simulink model "npc_controller"  (R2022a)
settings: Solver=FixedStepDiscrete  StartTime=0.0  StopTime=20  RelTol=1e-3  EnableMultiTasking=on
undefined symbols (not defined in the file): CAN_O_INT, CANA_BASE, Down, GPTRIP1SEL, GPTRIP2SEL, GPTRIP3SEL, Tsw, TZ1, TZ2, TZ3, Up
libraries: simulink x147, hdlsllib x90, c2802xlib x34, c2837xDlib x20, c280xlib x12, canmsglib x9, c2838xlib x8, idelinklib_common x3, c2806xlib x2, slpidlib x2, c28004xlib x2, c281xlib x2
(part 2 of 42)

== system npc_controller/CONTROL/CONTROL ==
  adc_in : Inport  OutDataTypeStr=Bus: adc_rect
  control_en1 : Inport  Port=2
  ref1 : Inport  Port=3
  angle1 : Inport  Port=4
  pol_pha1 : Inport  Port=5
  pol_phb1 : Inport  Port=6
  pol_phc1 : Inport  Port=7
  pha_en1 : Inport  Port=8
  phb_en1 : Inport  Port=9
  phc_en1 : Inport  Port=10
  pfc_ok2 : Inport  Port=11  OutDataTypeStr=boolean
  Trigger : TriggerPort  TriggerType=function-call  VariantControl=Variant  PortDimensions=1
  Data Store Read : DataStoreRead  DataStoreName=u8PriFutEnable  IndexOptions=Index vector (dialog)  Indices=1  OutputSizes=1
  If : If  IfExpression=u1 == 0
  false : Subsystem  TreatAsAtomicUnit=on
  sim_cmp1 : Outport
  Vpk : Outport  Port=2
  wires:
  If/1 -> false/Action
  Data Store Read/1 -> If/1
  adc_in/1 -> false/1(adc_in)
  control_en1/1 -> false/2(control_en1)
  ref1/1 -> false/3(ref1)
  false/1(sim_cmp1) -> sim_cmp1/1
  angle1/1 -> false/4(angle1)
  pol_pha1/1 -> false/5(pol_pha1)
  pol_phb1/1 -> false/6(pol_phb1)
  pol_phc1/1 -> false/7(pol_phc1)
  pha_en1/1 -> false/8(pha_en1)
  phb_en1/1 -> false/9(phb_en1)
  phc_en1/1 -> false/10(phc_en1)
  false/2(Vpk) -> Vpk/1
  pfc_ok2/1 -> false/11(pfc_ok2)

== system npc_controller/CONTROL/GET_ADC ==
  note: actual to vadc:
      | va               0.001799
      | vb               "
      | vc               "
      | vbulk          0.003623
      | vmid           0.006453
      | vaux           N/A
      |
      | icsa            0.019524
      | icsb            "
      | icsc            "
      | iphasea      0.02
      | iphaseb      "
      | iphasec      "
      |
      | tmp_mux    -
  adc_in : Inport
  Trigger : TriggerPort  TriggerType=function-call  VariantControl=Variant  PortDimensions=1
  ADC : Subsystem  Variant=on
  adc_out : Outport
  adc_rect : Outport  Port=2
  wires:
  adc_in/1 -> ADC/1(adc_in)
  ADC/1(adc_out) -> adc_out/1
  ADC/2(adc_rect) -> adc_rect/1

== system npc_controller/CONTROL/GPIO_HIGH ==
  Trigger : TriggerPort  TriggerType=function-call  VariantControl=Variant  PortDimensions=1
  Constant1 : Constant  Commented=on  OutDataTypeStr=single
  GPIO85_pin86 : c2837xDlib/Digital Output  Commented=on  GPIO_Number=GPIO80~GPIO87  GPIO_Bit0=off  GPIO_BIT0_Toggle=off  GPIO_Bit1=off  GPIO_BIT1_Toggle=off  GPIO_Bit2=off  GPIO_BIT2_Toggle=off  GPIO_Bit3=off  GPIO_BIT3_Toggle=off  GPIO_Bit4=off  GPIO_BIT4_Toggle=off  GPIO_Bit5=on  GPIO_BIT5_Toggle=off  GPIO_Bit6=off  GPIO_BIT6_Toggle=off  GPIO_Bit7=off  GPIO_BIT7_Toggle=off
      settings: SourceProductBaseCode=TIC2000
  wires:
  Constant1/1 -> GPIO85_pin86/1

== system npc_controller/CONTROL/GPIO_LOW ==
  Trigger : TriggerPort  TriggerType=function-call  VariantControl=Variant  PortDimensions=1
  Constant1 : Constant  Commented=on  Value=0  OutDataTypeStr=single
  GPIO85_pin86 : c2837xDlib/Digital Output  Commented=on  GPIO_Number=GPIO80~GPIO87  GPIO_Bit0=off  GPIO_BIT0_Toggle=off  GPIO_Bit1=off  GPIO_BIT1_Toggle=off  GPIO_Bit2=off  GPIO_BIT2_Toggle=off  GPIO_Bit3=off  GPIO_BIT3_Toggle=off  GPIO_Bit4=off  GPIO_BIT4_Toggle=off  GPIO_Bit5=on  GPIO_BIT5_Toggle=off  GPIO_Bit6=off  GPIO_BIT6_Toggle=off  GPIO_Bit7=off  GPIO_BIT7_Toggle=off
      settings: SourceProductBaseCode=TIC2000
  wires:
  Constant1/1 -> GPIO85_pin86/1

== system npc_controller/CONTROL/POLARITY ==
  note: Note:
      | 0 - pos
      | 1 - neg
  adc_in : Inport  OutDataTypeStr=Bus: adc
  Trigger : TriggerPort  TriggerType=function-call  VariantControl=Variant  PortDimensions=1
  Bus Selector : BusSelector  OutputSignals=va,vb,vc,ia,ib,ic,vbulk,vmid
  Constant : Constant  Value=0  OutDataTypeStr=single  SampleTime=-1
  Constant1 : Constant  Value=0  OutDataTypeStr=single  SampleTime=-1
  Constant2 : Constant  Value=0  OutDataTypeStr=single  SampleTime=-1
  GreaterThan : RelationalOperator  Operator=<  OutDataTypeStr=boolean  RndMeth=Simplest  InputSameDT=off
  GreaterThan1 : RelationalOperator  Operator=<  OutDataTypeStr=boolean  RndMeth=Simplest  InputSameDT=off
  GreaterThan2 : RelationalOperator  Operator=<  OutDataTypeStr=boolean  RndMeth=Simplest  InputSameDT=off
  Mux : Mux  Inputs=3
  PLL_Block1 : Subsystem  Commented=on  TreatAsAtomicUnit=on
      settings: RTWFcnNameOpts=Use subsystem name
  Scope : Scope  NumInputPorts=2
  Scope4 : Scope  Commented=on  NumInputPorts=4
  pol_pha : Outport
  pol_phb : Outport  Port=2
  pol_phc : Outport  Port=3
  wires:
  GreaterThan1/1 -> pol_phb/1
  GreaterThan/1 -> Scope/2, pol_pha/1
  adc_in/1 -> Bus Selector/1
  Bus Selector/1 -> [van]  "<va>"
  Bus Selector/3 -> [vcn]  "<vc>"
  Bus Selector/2 -> [vbn]  "<vb>"
  Constant/1 -> GreaterThan/2
  [van] -> Scope/1, GreaterThan/1
  GreaterThan2/1 -> pol_phc/1
  Constant1/1 -> GreaterThan1/2
  Constant2/1 -> GreaterThan2/2
  [vcn] -> GreaterThan2/1
  [vbn] -> GreaterThan1/1
  [van] -> Scope4/4
  [vbn] -> Scope4/2
  [van] -> Mux/3
  Mux/1 -> PLL_Block1/1(abc)
  [vcn] -> Scope4/3
  [vcn] -> Mux/2
  [vbn] -> Mux/1
  PLL_Block1/1(theta) -> Scope4/1  "va"

== system npc_controller/CONTROL/STATE-MACHINE ==
  note: States:
      | 0 - Calibraiton
      | 1 - Fault
      | 2 - FUT mode
      | 3 - NA
      | 4 - Control ON
      | 5 - Burst mode
      | 6 - PFC_EN Low
      | 7 - AC_OK Low
  note: 1 - Leg A
      | 2 - Leg B
      | 3 - Leg C
      | 4 - All legs
  note: 0 - Three phase
      | 1 - Single phase
  adc_out : Inport
  Vpk : Inport  Port=2
  Trigger : TriggerPort  TriggerType=function-call  VariantControl=Variant  PortDimensions=1
  Add : Sum  Commented=on  Inputs=+-  AccumDataTypeStr=single  OutDataTypeStr=single
  Bus Selector : BusSelector  OutputSignals=va,vb,vc,ia,ib,ic,vbulk,vmid
  CPU_CONTROL_100_A2_precharge_pfc_ok2 : Stateflow chart  Commented=on  TreatAsAtomicUnit=on
  CPU_CONTROL_200_A2_precharge_pfc_ok2 : Stateflow chart  Commented=on  TreatAsAtomicUnit=on
  CPU_CONTROL_200_A2_precharge_pfc_ok2_OL SS : Stateflow chart  Commented=on  TreatAsAtomicUnit=on
  CPU_CONTROL_200_A2_precharge_pfc_ok2_OL SS1 : Stateflow chart  Commented=on  TreatAsAtomicUnit=on
  CPU_CONTROL_200_Vpk : Stateflow chart  Commented=on  TreatAsAtomicUnit=on
  CPU_CONTROL_400 : Stateflow chart  Commented=on  TreatAsAtomicUnit=on
  CPU_CONTROL_400_A2_precharge_pfc_ok2_OL SS : Stateflow chart  Commented=on  TreatAsAtomicUnit=on
  CPU_CONTROL_750_A2_precharge_pfc_ok1 : Stateflow chart  Commented=on  TreatAsAtomicUnit=on
  CPU_CONTROL_750_A2_precharge_pfc_ok2_OL SS1 : Stateflow chart  Commented=on  TreatAsAtomicUnit=on
  CPU_CONTROL_750_A2_precharge_pfc_ok2_OL SS2 : Stateflow chart  TreatAsAtomicUnit=on
  CPU_CONTROL_750_Vpk : Stateflow chart  Commented=on  TreatAsAtomicUnit=on
  CPU_CONTROL_750_precharge_pfc_ok2 : Stateflow chart  Commented=on  TreatAsAtomicUnit=on
  Cast To Single : DataTypeConversion  Commented=on  OutDataTypeStr=uint16  SaturateOnIntegerOverflow=off  RndMeth=Floor
  Cast To Single1 : DataTypeConversion  Commented=on  OutDataTypeStr=single  SaturateOnIntegerOverflow=off  RndMeth=Floor
  Cast To Single2 : DataTypeConversion  OutDataTypeStr=single  SaturateOnIntegerOverflow=off  RndMeth=Floor
  Cast To Single3 : DataTypeConversion  Commented=on  OutDataTypeStr=single  SaturateOnIntegerOverflow=off  RndMeth=Floor
  Constant : Constant  OutDataTypeStr=boolean
  Constant2 : Constant  Commented=on  Value=200  OutDataTypeStr=single
  DAC : c2837xDlib/DAC  Commented=on  channel=B  saturate=on
      settings: SourceProductBaseCode=TIC2000
  Data Store Read : DataStoreRead  Commented=on  DataStoreName=debug_en  IndexOptions=Index vector (dialog)  Indices=1  OutputSizes=1
  Data Store Read1 : DataStoreRead  DataStoreName=u8PriFutEnable  IndexOptions=Index vector (dialog)  Indices=1  OutputSizes=1
  Data Store Read2 : DataStoreRead  DataStoreName=u8GridPhaseType  IndexOptions=Index vector (dialog)  Indices=1  OutputSizes=1
  Data Store Read3 : DataStoreRead  DataStoreName=u8SinglePhaseLeg  IndexOptions=Index vector (dialog)  Indices=1  OutputSizes=1
  Data Store Read4 : DataStoreRead  DataStoreName=pfc_en  IndexOptions=Index vector (dialog)  Indices=1  OutputSizes=1
  Data Store Read5 : DataStoreRead  DataStoreName=rms_vc  IndexOptions=Index vector (dialog)  Indices=1  OutputSizes=1
  Data Store Write : DataStoreWrite  DataStoreName=u16Debug1  IndexOptions=Index vector (dialog)  Indices=1  OutputSizes=1
  Data Store Write12 : DataStoreWrite  DataStoreName=relay_ctrl  IndexOptions=Index vector (dialog)  Indices=1  OutputSizes=1
  Data Store Write13 : DataStoreWrite  DataStoreName=pfc_ok  IndexOptions=Index vector (dialog)  Indices=1  OutputSizes=1
  Data Store Write3 : DataStoreWrite  DataStoreName=ac_ok  IndexOptions=Index vector (dialog)  Indices=1  OutputSizes=1
  Data Store Write4 : DataStoreWrite  DataStoreName=pfc_en  IndexOptions=Index vector (dialog)  Indices=1  OutputSizes=1
  Data Store Write5 : DataStoreWrite  Commented=on  DataStoreName=Vbulk_Ref  IndexOptions=Index vector (dialog)  Indices=1  OutputSizes=1
  Digital Output : c2837xDlib/Digital Output  Commented=on  GPIO_Number=GPIO136~GPIO143  GPIO_Bit0=off  GPIO_BIT0_Toggle=off  GPIO_Bit1=off  GPIO_BIT1_Toggle=off  GPIO_Bit2=off  GPIO_BIT2_Toggle=off  GPIO_Bit3=on  GPIO_BIT3_Toggle=off  GPIO_Bit4=off  GPIO_BIT4_Toggle=off  GPIO_Bit5=off  GPIO_BIT5_Toggle=off  GPIO_Bit6=off  GPIO_BIT6_Toggle=off  GPIO_Bit7=off  GPIO_BIT7_Toggle=off
      settings: SourceProductBaseCode=TIC2000
  Gain : Gain  Commented=on  Gain=4095/831.7167
  Gain1 : Gain  Commented=on  Gain=2000  ParamDataTypeStr=single  OutDataTypeStr=single
  Gain2 : Gain  Gain=500  ParamDataTypeStr=single  OutDataTypeStr=single
  Gain3 : Gain  Gain=1.414  OutDataTypeStr=single
  If : If  Commented=on  IfExpression=u1 == 0
  If Action Subsystem : Subsystem  Commented=on  TreatAsAtomicUnit=on
  If Action Subsystem1 : Subsystem  Commented=on  TreatAsAtomicUnit=on
  Merge : Merge  Commented=on
  NOT : Logic  Operator=NOT  IconShape=distinctive  AllPortsSameDT=off  OutDataTypeStr=boolean
  PFC_EN_GPIO60 : c2837xDlib/Digital Input  GPIO_Number=GPIO56~GPIO63  GPIO_Bit0=off  GPIO_Bit1=off  GPIO_Bit2=off  GPIO_Bit3=off  GPIO_Bit4=on  GPIO_Bit5=off  GPIO_Bit6=off  GPIO_Bit7=off  sampleTime=-1  dataType=auto  GPIO_Bit0_Qualification=Sync to SYSCLKOUT  GPIO_Bit1_Qualification=Sync to SYSCLKOUT  GPIO_Bit2_Qualification=Sync to SYSCLKOUT  GPIO_Bit3_Qualification=Sync to SYSCLKOUT  GPIO_Bit4_Qualification=Sync to SYSCLKOUT  GPIO_Bit5_Qualification=Sync to SYSCLKOUT  GPIO_Bit6_Qualification=Sync to SYSCLKOUT  GPIO_Bit7_Qualification=Sync to SYSCLKOUT  Qualification_Period=-1
      settings: SourceProductBaseCode=TIC2000
  PLL : Subsystem  Commented=on
  Sin2 : Trigonometry  Commented=on  OutputSignalType=real
  Subsystem1 : Subsystem  Commented=on
  Update_PFC_EN : Subsystem
  calib_ok : Outport
  control_en : Outport  Port=2
  burst_en : Outport  Port=3
  eoss : Outport  Port=4
  ref : Outport  Port=5
  mag : Outport  Port=6
  angle : Outport  Port=7
  freq : Outport  Port=8
  va_seq : Outport  Port=9
  vb_seq : Outport  Port=10
  vc_seq : Outport  Port=11
  pha_en : Outport  Port=12
  phb_en : Outport  Port=13
  phc_en : Outport  Port=14
  pfc_ok1 : Outport  Port=15
  wires:
  CPU_CONTROL_750_A2_precharge_pfc_ok2_OL SS2/6(ref) -> ref/1, Cast To Single/1
  adc_out/1 -> Bus Selector/1
  Bus Selector/7 -> CPU_CONTROL_750_A2_precharge_pfc_ok2_OL SS2/7(vbulk)  "<vbulk>"
  Bus Selector/1 -> CPU_CONTROL_750_A2_precharge_pfc_ok2_OL SS2/1(van)  "<va>"
  Bus Selector/2 -> CPU_CONTROL_750_A2_precharge_pfc_ok2_OL SS2/2(vbn)  "<vb>"
  Bus Selector/3 -> CPU_CONTROL_750_A2_precharge_pfc_ok2_OL SS2/3(vcn)  "<vc>"
  CPU_CONTROL_750_A2_precharge_pfc_ok2_OL SS2/3(control_en) -> control_en/1
  CPU_CONTROL_750_A2_precharge_pfc_ok2_OL SS2/4(burst_en) -> burst_en/1
  CPU_CONTROL_750_A2_precharge_pfc_ok2_OL SS2/5(eoss) -> eoss/1
  Bus Selector/4 -> CPU_CONTROL_750_A2_precharge_pfc_ok2_OL SS2/4(ia)  "<ia>"
  Bus Selector/5 -> CPU_CONTROL_750_A2_precharge_pfc_ok2_OL SS2/5(ib)  "<ib>"
  Bus Selector/6 -> CPU_CONTROL_750_A2_precharge_pfc_ok2_OL SS2/6(ic)  "<ic>"
  Sin2/1 -> Subsystem1/1(adc)
  Add/1 -> PLL/1(vxn)
  Cast To Single3/1 -> Add/1
  Merge/1 -> Add/2
  PLL/2(angle) -> Sin2/1
  Subsystem1/1(adc_rect) -> angle/1  "va"
  CPU_CONTROL_750_A2_precharge_pfc_ok2_OL SS2/2(calib_ok) -> calib_ok/1
  If/1 -> If Action Subsystem1/Action
  If Action Subsystem/1(Out1) -> Merge/2
  If Action Subsystem1/1(Out1) -> Merge/1
  If/2 -> If Action Subsystem/Action
  Data Store Read/1 -> ?
  Data Store Read1/1 -> CPU_CONTROL_750_A2_precharge_pfc_ok2_OL SS2/8(fut_en_req)
  CPU_CONTROL_750_A2_precharge_pfc_ok2_OL SS2/10(pha_en) -> va_seq/1, pha_en/1
  CPU_CONTROL_750_A2_precharge_pfc_ok2_OL SS2/11(phb_en) -> vb_seq/1, phb_en/1
  CPU_CONTROL_750_A2_precharge_pfc_ok2_OL SS2/12(phc_en) -> vc_seq/1, phc_en/1
  CPU_CONTROL_750_A2_precharge_pfc_ok2_OL SS2/1(state) -> Data Store Write/1, Cast To Single2/1
  Cast To Single/1 -> ?
  Data Store Read2/1 -> CPU_CONTROL_750_A2_precharge_pfc_ok2_OL SS2/9(grid_config_req)
  Data Store Read3/1 -> CPU_CONTROL_750_A2_precharge_pfc_ok2_OL SS2/10(singleph_config_req)
  Cast To Single1/1 -> Gain1/1
  Cast To Single2/1 -> Gain2/1
  Gain2/1 -> ?
  Data Store Read5/1 -> Gain3/1
  CPU_CONTROL_750_A2_precharge_pfc_ok2_OL SS2/13(pfc_ok) -> pfc_ok1/1, Data Store Write13/1
  CPU_CONTROL_750_A2_precharge_pfc_ok2_OL SS2/14(relay_ctrl) -> Data Store Write12/1
  Data Store Read4/1 -> CPU_CONTROL_750_A2_precharge_pfc_ok2_OL SS2/12(pfc_en)
  CPU_CONTROL_750_A2_precharge_pfc_ok2_OL SS2/15(tfv_v_UvpOvp) -> NOT/1
  NOT/1 -> Data Store Write3/1
  Update_PFC_EN/1(Dig_Input_State) -> Digital Output/1, Data Store Write4/1
  Gain/1 -> Data Store Write5/1
  Constant2/1 -> Gain/1
  Gain3/1 -> CPU_CONTROL_750_A2_precharge_pfc_ok2_OL SS2/11(Vpk)
  Gain1/1 -> DAC/1
  Constant/1 -> Update_PFC_EN/1(Dig_Input)

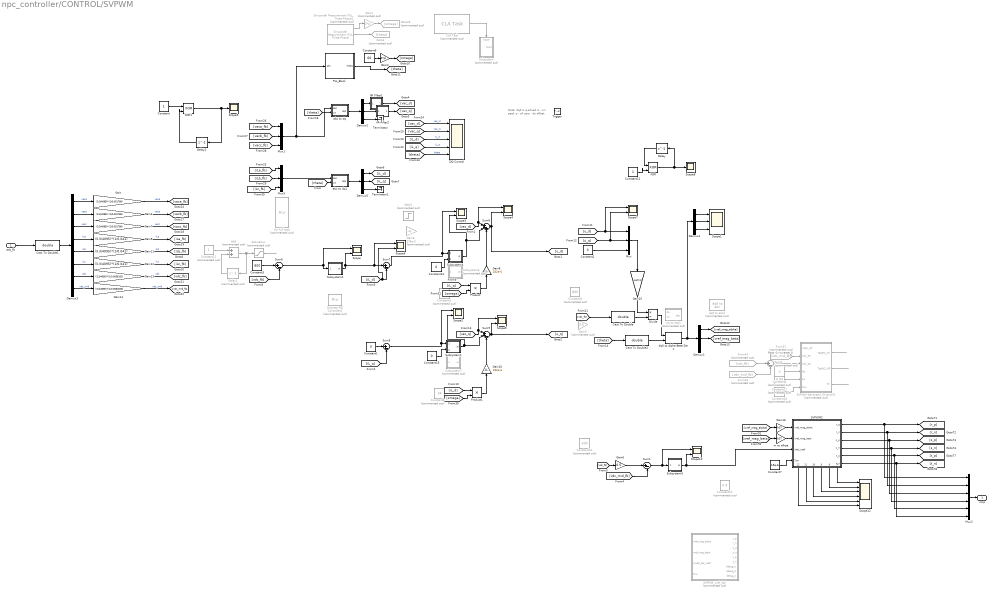
== system npc_controller/CONTROL/SVPWM ==
  note: Note: dq0 is q-alined
      | d - vin peak
      | q - pf
      | zero - dc offset
  note: Rect -1, inverter 0
  adc_fb : Inport
  Trigger : TriggerPort  TriggerType=function-call  VariantControl=Variant  PortDimensions=1
  Add : Sum  Commented=on
  CLA Task : c2806xlib/CLA Task  Commented=on  taskNumber=1  intSource=Software  wait=off  sampleTime=-1  claType=0  softTrigSelected=1  enableInterrupt=on
      settings: SourceProductName=Embedded Coder Support Package for Texas Instruments C2000 Processors
  Cast To Double : DataTypeConversion  OutDataTypeStr=double  SaturateOnIntegerOverflow=off  RndMeth=Floor
  Cast To Double1 : DataTypeConversion  OutDataTypeStr=double  SaturateOnIntegerOverflow=off  RndMeth=Floor
  Cast To Double2 : DataTypeConversion  OutDataTypeStr=double  SaturateOnIntegerOverflow=off  RndMeth=Floor
  Constant : Constant
  Constant{1..2,13,15} (4 alike) : Constant  Value=0
  Constant10 : Constant  Commented=on  Value=0.9
  Constant11 : Constant  Commented=on
  Constant12 : Constant
  Constant14 : Constant  Commented=on  Value=400
  Constant17 : Constant  Commented=on  Value=0.04
  Constant18 : Constant  Commented=on  Value=65e3
  Constant3 : Constant  Value=800
  Constant4 : Constant  Commented=on  Value=-1
  Constant5 : Constant  Commented=on  Value=34
  Constant6 : Constant  Value=60
  Constant7 : Constant  Value=15e-6
  Constant8 : Constant  Commented=on  Value=34
  Constant9 : Constant  Commented=on  Value=800
  DQ Control : Scope  NumInputPorts=5
  Delay : Delay  DelayLength=1
  Delay1 : Delay  Commented=on  DelayLength=1
  Delay2 : Delay  DelayLength=1
  Demux{1..2,4..5} (4 alike) : Demux  Outputs=3
  Demux3 : Demux  Outputs=8
  Discrete PID Controller2 : slpidlib/PID Controller  Commented=on  Controller=PI  Form=Ideal  TimeDomain=Discrete-time  UseExternalTs=off  SampleTime=-1  IntegratorMethod=Forward Euler  FilterMethod=Forward Euler  ControllerParametersSource=internal  P=0.611  I=33.333  UseKiTs=off  D=0  N=100  UseFilter=on  TunerSelectOption=Transfer Function Based (PID Tuner App)  InitialConditionSource=internal  InitialConditionForIntegrator=22  InitialConditionForFilter=0  DifferentiatorICPrevScaledInput=0  ExternalReset=none  TrackingMode=off  Kt=1  LimitOutput=on  SatLimitsSource=internal  UpperSaturationLimit=36  LowerSaturationLimit=-36  LinearizeAsGain=off  AntiWindupMode=none  Kb=1  POutMin=[]  POutMax=[]  IOutMin=[]  IOutMax=[]  DOutMin=[]  DOutMax=[]  NOutMin=[]  NOutMax=[]  SumOutMin=[]  SumOutMax=[]  SaturationOutMin=[]  SaturationOutMax=[]  PParamMin=[]  PParamMax=[]  IParamMin=[]  IParamMax=[]  DParamMin=[]  DParamMax=[]  NParamMin=[]  NParamMax=[]  KbParamMin=[]  KbParamMax=[]  KtParamMin=[]  KtParamMax=[]  KbOutMin=[]  KbOutMax=[]  KtOutMin=[]  KtOutMax=[]  IntegratorOutMin=[]  IntegratorOutMax=[]  FilterOutMin=[]  FilterOutMax=[]  SumI1OutMin=[]  SumI1OutMax=[]  SumI2OutMin=[]  SumI2OutMax=[]  SumI3OutMin=[]  SumI3OutMax=[]  SumI4OutMin=[]  SumI4OutMax=[]  SumDOutMin=[]  SumDOutMax=[]  DifferentiatorOutMin=[]  DifferentiatorOutMax=[]  FilterDiffOutCoefMin=[]  FilterDiffOutCoefMax=[]  ReciprocalOutMin=[]  ReciprocalOutMax=[]  SumDenOutMin=[]  SumDenOutMax=[]  SumNumOutMin=[]  SumNumOutMax=[]  DivideOutMin=[]  DivideOutMax=[]  UdiffTsProdOutMin=[]  UdiffTsProdOutMax=[]  NTsProdOutMin=[]  NTsProdOutMax=[]  UintegralTsProdOutMin=[]  UintegralTsProdOutMax=[]  UngainTsProdOutMin=[]  UngainTsProdOutMax=[]  IntegratorContinuousStateAttributes=''  IntegratorStateMustResolveToSignalObject=off  IntegratorRTWStateStorageClass=Auto  FilterContinuousStateAttributes=''  FilterStateMustResolveToSignalObject=off  FilterRTWStateStorageClass=Auto  ParallelPVariant=Passthrough  IdealPVariant=InternalParameters  IVariant=InternalParameters  DVariant=Disabled  IntegratorVariant=Discrete  SatVariant=Enabled  AWVariant=Passthrough  PCopyVariant=Disabled  TRVariant=Disabled  FdbkBlocksVariant=Forward  IdealPFdbkVariant=Disabled  SatFdbkVariant=Disabled  DerivativeFilterVariant=Disabled  NVariant=Disabled  NCopyVariant=Disabled_SignalSpec  FilterICVariant=Disabled  IntegratorICVariant=InternalICs  ExternalResetVariant=Disabled  TRSumVariant=Passthrough  SumFdbkVariant=Disabled  SumVariant=Sum_PI  TsampFilterVariant=InternalTs  TsampNgainVariant=Passthrough  TsampIntegralVariant=Passthrough  ExternalSaturationOutDataTypeStr=Inherit: Same as second input  aMode=0
  Divide : Product  Inputs=*/
  From37 : From  Commented=on  GotoTag=vdc_mid_fb
  From42 : From  Commented=on  GotoTag=vdc_mid_fb
  From43 : From  Commented=on  GotoTag=vdc_fb
  Gain : Gain  Gain=(3.3/4095)*(1/0.001798)
  Gain1 : Gain  Commented=on  Gain=2*pi
  Gain10 : Gain  Gain=182e-6
  Gain11 : Gain  Gain=(3.3/4095)*(1/0.041)
  Gain12 : Gain  Gain=(3.3/4095)*(1/0.041)
  Gain13 : Gain  Gain=(3.3/4095)*(1/0.0036102)
  Gain14 : Gain  Gain=(3.3/4095)*(1/0.0064528)
  Gain15 : Gain  Gain=sqrt(3)
  Gain16 : Gain  Gain=0.57
  Gain2 : Gain  Gain=2*pi
  Gain3 : Gain  Commented=on  Gain=2*5e-3
  Gain4 : Gain  Gain=(3.3/4095)*(1/0.001798)
  Gain5 : Gain  Commented=on  Gain=0.5
  Gain6 : Gain  Gain=0.5
  Gain7 : Gain  Gain=(3.3/4095)*(1/0.001798)
  Gain8 : Gain  Gain=182e-6
  Gain9 : Gain  Gain=(3.3/4095)*(1/0.041)
  Goto25 : Goto  Commented=on  GotoTag=omega
  Goto3 : Goto  Commented=on  GotoTag=theta
  IIR Filter1 : Subsystem
  IIR Filter2 : Subsystem
  Mux : Mux  Inputs=3
  Mux1 : Mux  Inputs=3
  Mux2 : Mux  Inputs=6
  Mux5 : Mux  Inputs=3
  PLL_Block : Subsystem  TreatAsAtomicUnit=on
      settings: RTWFcnNameOpts=Use subsystem name
  Product : Product
  Product1 : Product
  SVPWM Generator (3-Level)1 : Subsystem  Commented=on
  SVPWM2 : Stateflow chart  TreatAsAtomicUnit=on
      settings: PortSchema="{\"entries\":[{\"content\":{\"sides\":[{\"content\":{\"connectorIds\":[\"In1\",\"In2\",\"In3\",\"In4\"]},\"type\":\"ConnectorPlacement.EquallySpacedRectSide\",\"uuid\":\"7e4e3e66-8524-4070-820d-e987ee6a426b\"},{\"content\":{\"connectorIds\":[\"Out1\",\"Out2\",\"Out3\",\"Out4\",\"Out5\",\"Out6\"],\"side\":\"RIGHT\"},\"type\":\"ConnectorPlacement.EquallySpacedRectSide\",\"uuid\":\"f5c3bbe2-d26b-4560-8bc2-49e1d2ba310c\"},{\"content\":{\"connectorIds\":[],\"side\":\"TOP\"},\"type\":\"ConnectorPlacement.EquallySpacedRectSide\",\"uuid\":\"83d02455-8012-4bd6-97d4-4ddb2b0da207\"},{\"content\":{\"connectorIds\":[\"Out12\",\"Out11\",\"Out10\",\"Out9\",\"Out8\",\"Out7\"],\"side\":\"BOTTOM\"},\"type\":\"ConnectorPlacement.EquallySpacedRectSide\",\"uuid\":\"82480829-29a6-4c64-92d2-d0891a7cd2c4\"},{\"content\":{\"connectorIds\":[],\"side\":\"HIDDEN\"},\"type\":\"ConnectorPlacement.EquallySpacedRectSide\",\"uuid\":\"daebbe37-e4fd-4cc7-9cba-3ce58bd0f8bb\"}]},\"type\":\"ConnectorPlacement.EquallySpacedConnector\",\"uuid\":\"3945a731-6436-4370-b05f-e1cd706c7526\"}],\"packageUris\":[\"http://schema.mathworks.com/mf0/Connector/R2020b\"],\"version\":\"1.0\"}"
  SVPWM_with_bal : Stateflow chart  Commented=on  TreatAsAtomicUnit=on
  Saturation : Saturate  Commented=on  UpperLimit=800  LowerLimit=0
  Scope{,2..7,10} (8 alike) : Scope  NumInputPorts=2
  Scope1 : Scope  NumInputPorts=3
  Scope12 : Scope  NumInputPorts=6
  Scope8 : Scope
  Scope9 : Scope
  "Sinusoidal Measurement (PLL, Three-Phase)1" : eeSinusoidalMeasurementV2/Sinusoidal Measurement (PLL, Three-Phase)  Commented=on  Kp_LF=2  Ki_LF=20  F0=60  Theta0=0  Ts=-1
      settings: SourceProductBaseCode=PS
  Step2 : Step  Commented=on  Time=0.07  Before=10  After=2*5e-3  SampleTime=0
  Subsystem : Subsystem  Commented=on
  Subsystem1 : Subsystem
      mask Display: disp('PID(z)')
  Subsystem2 : Subsystem
      mask Display: disp('PID(z)')
  Subsystem4 : Subsystem
      mask Display: disp('PID(z)')
  Subsystem5 : Subsystem
      mask Display: disp('PID(z)')
  Subsystem6 : Subsystem  Commented=on
      mask Display: disp('PID(z)')
  Subsystem7 : Subsystem  Commented=on
      mask Display: disp('PID(z)')
  Sum{1,5..7} (4 alike) : Sum  Inputs=|+-
  Sum2 : Sum  Commented=on  Inputs=|+-
  Sum8 : Sum  Inputs=|+-+
  Sum9 : Sum  Inputs=|+--
  Terminator : Terminator
  Terminator1 : Terminator
  XOR : Logic  Operator=XOR  IconShape=distinctive  AllPortsSameDT=off  OutDataTypeStr=boolean
  XOR1 : Logic  Operator=XOR  IconShape=distinctive  AllPortsSameDT=off  OutDataTypeStr=boolean
  abc to dq : Subsystem
  abc to dq1 : Subsystem
  dq to abc2 : Subsystem  Commented=on
  dq0 to Alpha-Beta-Zero : spsdq0toAlphaBetaZeroLib/dq0 to Alpha-Beta-Zero  Alignment=90 degrees behind phase A axis
      settings: SourceProductBaseCode=PS
  dq0 to abc1 : spsdq0toabcLib/dq0 to abc  Commented=on  Alignment=90 degrees behind phase A axis
  for full load : slpidlib/PID Controller  Commented=on  Controller=PI  Form=Parallel  TimeDomain=Discrete-time  UseExternalTs=off  SampleTime=-1  IntegratorMethod=Forward Euler  FilterMethod=Forward Euler  ControllerParametersSource=internal  P=10  I=10  UseKiTs=off  D=0  N=100  UseFilter=off  TunerSelectOption=Transfer Function Based (PID Tuner App)  InitialConditionSource=internal  InitialConditionForIntegrator=0  InitialConditionForFilter=0  DifferentiatorICPrevScaledInput=0  ExternalReset=none  TrackingMode=off  Kt=1  LimitOutput=on  SatLimitsSource=external  UpperSaturationLimit=450  LowerSaturationLimit=-450  LinearizeAsGain=on  AntiWindupMode=clamping  Kb=1  POutMin=[]  POutMax=[]  IOutMin=[]  IOutMax=[]  DOutMin=[]  DOutMax=[]  NOutMin=[]  NOutMax=[]  SumOutMin=[]  SumOutMax=[]  SaturationOutMin=[]  SaturationOutMax=[]  PParamMin=[]  PParamMax=[]  IParamMin=[]  IParamMax=[]  DParamMin=[]  DParamMax=[]  NParamMin=[]  NParamMax=[]  KbParamMin=[]  KbParamMax=[]  KtParamMin=[]  KtParamMax=[]  KbOutMin=[]  KbOutMax=[]  KtOutMin=[]  KtOutMax=[]  IntegratorOutMin=[]  IntegratorOutMax=[]  FilterOutMin=[]  FilterOutMax=[]  SumI1OutMin=[]  SumI1OutMax=[]  SumI2OutMin=[]  SumI2OutMax=[]  SumI3OutMin=[]  SumI3OutMax=[]  SumI4OutMin=[]  SumI4OutMax=[]  SumDOutMin=[]  SumDOutMax=[]  DifferentiatorOutMin=[]  DifferentiatorOutMax=[]  FilterDiffOutCoefMin=[]  FilterDiffOutCoefMax=[]  ReciprocalOutMin=[]  ReciprocalOutMax=[]  SumDenOutMin=[]  SumDenOutMax=[]  SumNumOutMin=[]  SumNumOutMax=[]  DivideOutMin=[]  DivideOutMax=[]  UdiffTsProdOutMin=[]  UdiffTsProdOutMax=[]  NTsProdOutMin=[]  NTsProdOutMax=[]  UintegralTsProdOutMin=[]  UintegralTsProdOutMax=[]  UngainTsProdOutMin=[]  UngainTsProdOutMax=[]  IntegratorContinuousStateAttributes=''  IntegratorStateMustResolveToSignalObject=off  IntegratorRTWStateStorageClass=Auto  FilterContinuousStateAttributes=''  FilterStateMustResolveToSignalObject=off  FilterRTWStateStorageClass=Auto  ParallelPVariant=InternalParameters  IdealPVariant=Disabled  IVariant=InternalParameters  DVariant=Disabled  IntegratorVariant=Discrete  SatVariant=External  AWVariant=DiscClampingParallel  PCopyVariant=Disabled  TRVariant=Disabled  FdbkBlocksVariant=Forward  IdealPFdbkVariant=Disabled  SatFdbkVariant=Disabled  DerivativeFilterVariant=Disabled  NVariant=Disabled  NCopyVariant=Disabled_SignalSpec  FilterICVariant=Disabled  IntegratorICVariant=InternalICs  ExternalResetVariant=Disabled  TRSumVariant=Passthrough  SumFdbkVariant=Disabled  SumVariant=Sum_PI  TsampFilterVariant=InternalTs  TsampNgainVariant=Passthrough  TsampIntegralVariant=Passthrough  ExternalSaturationOutDataTypeStr=Inherit: Same as second input  aMode=0
  m to alhpa : Gain  Gain=0.57
  cmp : Outport
  wires:
  CLA Task/1 -> Subsystem/Trigger
  IIR Filter2/1(y[n]) -> [vac_q]
  IIR Filter1/1(y[n]) -> [vac_d]
  Constant15/1 -> Subsystem1/2(disable)
  Constant13/1 -> Subsystem4/2(disable)
  m to alhpa/1 -> SVPWM2/2(vref_mag_beta)
  Gain16/1 -> SVPWM2/1(vref_mag_alpha)
  Gain15/1 -> Divide/1
  Subsystem5/1(pi) -> Scope10/2, SVPWM2/3(vbal_coef)
  [vdc_fb] -> Gain6/1
  Constant7/1 -> SVPWM2/4(Tsw)
  [vdc_fb] -> Cast To Double/1
  Saturation/1 -> ?
  Delay1/1 -> Add/2
  Add/1 -> Delay1/1, Saturation/1
  Constant11/1 -> Add/1
  SVPWM2/12(debug_f) -> Scope12/6
  SVPWM2/10(debug_d) -> Scope12/4
  SVPWM2/11(debug_e) -> Scope12/5
  SVPWM2/9(debug_c) -> Scope12/3
  SVPWM2/8(debug_b) -> Scope12/2
  SVPWM2/7(debug_a) -> Scope12/1
  Gain6/1 -> Sum1/1
  Sum1/1 -> Subsystem5/1(error), Scope10/1
  [vdc_mid_fb] -> Sum1/2
  Mux2/1 -> cmp/1
  Cast To Double2/1 -> dq0 to Alpha-Beta-Zero/2
  Demux1/2 -> [vref_mag_beta]
  Demux1/1 -> [vref_mag_alpha]
  SVPWM2/2(r_n) -> [r_n], Mux2/2
  SVPWM2/3(s_p) -> [s_p], Mux2/3
  SVPWM2/5(t_p) -> [t_p], Mux2/5
  SVPWM2/6(t_n) -> [t_n], Mux2/6
  SVPWM2/4(s_n) -> [s_n], Mux2/4
  SVPWM2/1(r_p) -> [r_p], Mux2/1
  [vref_mag_beta] -> m to alhpa/1
  [vref_mag_alpha] -> Gain16/1
  Constant6/1 -> Gain2/1
  PLL_Block/1(theta) -> [theta]
  Gain2/1 -> [omega]
  abc to dq/1(dq0) -> Demux2/1
  Demux3/5 -> Gain11/1  "iLb"
  Demux3/4 -> Gain9/1  "iLa"
  Demux3/3 -> Gain7/1  "vacc"
  Demux3/2 -> Gain4/1  "vacb"
  Demux3/6 -> Gain12/1  "iLc"
  Demux3/7 -> Gain13/1  "vdc"
  Demux3/8 -> Gain14/1  "vdc_mid"
  Demux3/1 -> Gain/1  "vaca"
  Delay2/1 -> XOR1/2
  XOR1/1 -> Delay2/1, Scope9/1
  Constant/1 -> XOR1/1
  Gain14/1 -> [vdc_mid_fb]  "vdc_mid"
  Gain13/1 -> [vdc_fb]  "vdc"
  Gain12/1 -> [iLc_fb]  "iLc"
  Gain11/1 -> [iLb_fb]  "iLb"
  Gain9/1 -> [iLa_fb]  "iLa"
  Gain7/1 -> [vacc_fb]  "vacc"
  Gain4/1 -> [vacb_fb]  "vacb"
  Gain/1 -> [vaca_fb]  "vaca"
  Cast To Double1/1 -> Demux3/1
  Cast To Double/1 -> Divide/2
  SVPWM Generator (3-Level)1/3(Sn) -> ?
  SVPWM Generator (3-Level)1/2(TgABC_Off) -> ?
  SVPWM Generator (3-Level)1/1(TgABC_On) -> ?
  Sum2/1 -> SVPWM Generator (3-Level)1/3(Vdc_0N)
  From42/1 -> Sum2/2
  From37/1 -> SVPWM Generator (3-Level)1/2(Vdc_P0)
  From43/1 -> Sum2/1
  Constant17/1 -> SVPWM Generator (3-Level)1/5(Kp)
  Constant4/1 -> SVPWM Generator (3-Level)1/4(Idc)
  Constant18/1 -> SVPWM Generator (3-Level)1/6(Fsw)
  Gain1/1 -> Goto25/1
  "Sinusoidal Measurement (PLL, Three-Phase)1"/1 -> Gain1/1
  adc_fb/1 -> Cast To Double1/1
  [iLa_fb] -> Mux5/1
  [iLc_fb] -> Mux5/3
  [iLb_fb] -> Mux5/2
  [vacb_fb] -> Mux1/2
  [vaca_fb] -> Mux1/1
  [vacc_fb] -> Mux1/3
  [vac_q] -> DQ Control/2  "vac_q"
  [theta] -> DQ Control/5  "theta"
  [vac_d] -> DQ Control/1  "vac_d"
  Demux5/3 -> Terminator1/1
  [iL_d] -> DQ Control/3  "iL_d"
  [iL_q] -> DQ Control/4  "iL_q"
  Mux1/1 -> abc to dq/1(abc), PLL_Block/1(abc)
  [theta] -> abc to dq/2(wt)
  Mux5/1 -> abc to dq1/1(abc)
  Demux2/2 -> IIR Filter2/1(x[n])
  Demux5/1 -> [iL_d]
  [theta] -> abc to dq1/2(wt)
  Demux2/1 -> IIR Filter1/1(x[n])
  Demux2/3 -> Terminator/1
  Demux5/2 -> [iL_q]
  "Sinusoidal Measurement (PLL, Three-Phase)1"/2 -> Goto3/1
  abc to dq1/1(dq0) -> Demux5/1
  Gain10/1 -> Sum9/3
  Gain8/1 -> Sum8/3
  Mux/1 -> Gain15/1
  Delay/1 -> XOR/1
  XOR/1 -> Scope8/1, Delay/1
  Constant12/1 -> XOR/2
  Divide/1 -> dq0 to Alpha-Beta-Zero/1
  Subsystem2/1(pi) -> Scope/2, Sum7/1, Scope6/1
  dq0 to Alpha-Beta-Zero/1 -> Demux1/1, Demux4/1
  [theta] -> Cast To Double2/1
  [omega] -> Product1/2
  [omega] -> Product/2
  Product1/1 -> Gain10/1
  Product/1 -> Gain8/1
  [iL_q] -> Product/1
  [iL_d] -> Product1/1
  Sum9/1 -> Scope5/2, [u_q]
  Sum8/1 -> Scope4/2, [u_d]
  Constant2/1 -> Mux/3
  Demux4/3 -> Scope1/3
  Demux4/2 -> Scope1/2
  Demux4/1 -> Scope1/1
  [iL_d] -> Sum7/2, Scope6/2
  Sum5/1 -> Scope2/1, Subsystem1/1(error)
  Constant1/1 -> Sum5/1
  [iL_q] -> Sum5/2
  [vac_q] -> Sum9/1, Scope5/1
  Constant3/1 -> Sum6/1
  Sum6/1 -> Scope/1, Subsystem2/1(error)
  Subsystem4/1(pi) -> Scope3/2, Sum8/2
  Sum7/1 -> Scope3/1, Subsystem4/1(error)
  Subsystem1/1(pi) -> Scope2/2, Sum9/2
  [vac_d] -> Sum8/1, Scope4/1
  [vdc_fb] -> Sum6/2
  [u_q] -> Mux/2, Scope7/2
  [u_d] -> Mux/1, Scope7/1

== system npc_controller/IDLE_AND_TIMER/codegen ==
  note: Pre-charge relay ON/OFF
  note: Note: relay bypass
  note: CAN Task called @ 50Hz
      | (Every 20mS)
  AC_OK_GPIO41 : c2838xlib/Digital Output  GPIO_Number=GPIO40~GPIO47  GPIO_Bit0=off  GPIO_BIT0_Toggle=off  GPIO_Bit1=on  GPIO_BIT1_Toggle=off  GPIO_Bit2=off  GPIO_BIT2_Toggle=off  GPIO_Bit3=off  GPIO_BIT3_Toggle=off  GPIO_Bit4=off  GPIO_BIT4_Toggle=off  GPIO_Bit5=off  GPIO_BIT5_Toggle=off  GPIO_Bit6=off  GPIO_BIT6_Toggle=off  GPIO_Bit7=off  GPIO_BIT7_Toggle=off
      settings: SourceProductBaseCode=TIC2000
  CAN_Task : Subsystem
  Chart1 : Stateflow chart  TreatAsAtomicUnit=on  SystemSampleTime=20e-3
  Constant : Constant  Commented=on  OutDataTypeStr=boolean  SampleTime=-1
  Constant2 : Constant  Commented=on  OutDataTypeStr=boolean
  Data Store Read : DataStoreRead  DataStoreName=relay_ctrl  IndexOptions=Index vector (dialog)  Indices=1  OutputSizes=1
  Data Store Read1 : DataStoreRead  DataStoreName=pfc_ok  IndexOptions=Index vector (dialog)  Indices=1  OutputSizes=1
  Data Store Read2 : DataStoreRead  DataStoreName=ac_ok  IndexOptions=Index vector (dialog)  Indices=1  OutputSizes=1
  Data Store Write12 : DataStoreWrite  Commented=on  DataStoreName=u16Debug5  IndexOptions=Index vector (dialog)  Indices=1  OutputSizes=1
  Data Store Write2 : DataStoreWrite  Commented=on  DataStoreName=u16Debug4  IndexOptions=Index vector (dialog)  Indices=1  OutputSizes=1
  IDLE : Subsystem
  INITIALIZATION : Subsystem
  Idle Task : idelinklib_common/Idle Task  tasknumbers=[1]  taskpriorities=100017  taskpreempts=[1]  showinput=off  simPriority=0
      settings: SourceProductBaseCode=ME
  Memory Copy : idelinklib_common/Memory Copy  Commented=on  copyFrom=Specified source code symbol  copyFromAddressSource=Specify via dialog  copyFromAddress=hex2dec('00001000')  copyFromSrcCode=&CpuSysRegs.RESC  dataTypeFrom=uint32  dataDimensionFrom=1  useOffsetFrom=off  offsetFromSrc=Specify via dialog  offsetFrom=0  strideFrom=1  copyTo=Output port  copyToAddressSource=Specify via dialog  copyToAddress=hex2dec('00002000')  copyToSrcCode=myVariableDst  dataTypeTo=uint16  useOffsetTo=off  offsetToSrc=Specify via dialog  offsetTo=0  strideTo=1  sampleTime=inf  useInitValue=off  initValueSrc=Specify constant value  initValue=1  initValueSrcCode=myInitValueVariable  useAsMask=off  maskOperator=bitwise AND  useTermValue=off  termValue=1  isRealtimeEnabled=off  emitCCBeforeWrite=off  CCBeforeWrite=/* Custom Code Before Write*/  emitCCAfterWrite=off  CCAfterWrite=/* Custom Code After Write*/  useDMACopy=off  enableBlockingMode=off
      settings: SourceProductBaseCode=ME
  PFC_OK_GPIO58 : c2838xlib/Digital Output  GPIO_Number=GPIO56~GPIO63  GPIO_Bit0=off  GPIO_BIT0_Toggle=off  GPIO_Bit1=off  GPIO_BIT1_Toggle=off  GPIO_Bit2=on  GPIO_BIT2_Toggle=off  GPIO_Bit3=off  GPIO_BIT3_Toggle=off  GPIO_Bit4=off  GPIO_BIT4_Toggle=off  GPIO_Bit5=off  GPIO_BIT5_Toggle=off  GPIO_Bit6=off  GPIO_BIT6_Toggle=off  GPIO_Bit7=off  GPIO_BIT7_Toggle=off
      settings: SourceProductBaseCode=TIC2000
  RELAY_GPIO4_EPWM3A : c2838xlib/Digital Output  Commented=on  GPIO_Number=GPIO0~GPIO7  GPIO_Bit0=off  GPIO_BIT0_Toggle=off  GPIO_Bit1=off  GPIO_BIT1_Toggle=off  GPIO_Bit2=off  GPIO_BIT2_Toggle=off  GPIO_Bit3=off  GPIO_BIT3_Toggle=off  GPIO_Bit4=on  GPIO_BIT4_Toggle=off  GPIO_Bit5=off  GPIO_BIT5_Toggle=off  GPIO_Bit6=off  GPIO_BIT6_Toggle=off  GPIO_Bit7=off  GPIO_BIT7_Toggle=off
      settings: SourceProductBaseCode=TIC2000
  RELAY_GPIO4_EPWM3A1 : c2838xlib/Digital Output  GPIO_Number=GPIO0~GPIO7  GPIO_Bit0=off  GPIO_BIT0_Toggle=off  GPIO_Bit1=off  GPIO_BIT1_Toggle=off  GPIO_Bit2=off  GPIO_BIT2_Toggle=off  GPIO_Bit3=off  GPIO_BIT3_Toggle=off  GPIO_Bit4=on  GPIO_BIT4_Toggle=off  GPIO_Bit5=off  GPIO_BIT5_Toggle=off  GPIO_Bit6=off  GPIO_BIT6_Toggle=off  GPIO_Bit7=off  GPIO_BIT7_Toggle=off
      settings: SourceProductBaseCode=TIC2000
  TIMER_100MS : Subsystem  Commented=on  TreatAsAtomicUnit=on  ScheduleAs=Periodic partition  PartitionName=timer_100ms  SystemSampleTime=100e-3
      settings: RTWFcnNameOpts=Use subsystem name  RTWFileNameOpts=Use subsystem name
  TIMER_1MS : Subsystem  Variant=on
  u32 Data to 2xu16 : Subsystem  Commented=on
  wires:
  Idle Task/1 -> IDLE/Trigger
  Chart1/1(sim_control()) -> CAN_Task/Trigger
  Constant/1 -> RELAY_GPIO4_EPWM3A/1
  Data Store Read/1 -> RELAY_GPIO4_EPWM3A1/1
  Data Store Read1/1 -> PFC_OK_GPIO58/1
  Data Store Read2/1 -> AC_OK_GPIO41/1
  Memory Copy/1 -> u32 Data to 2xu16/1(u32 Data)
  u32 Data to 2xu16/1(u16Lsb) -> Data Store Write2/1
  u32 Data to 2xu16/2(u16Msb) -> Data Store Write12/1

== system npc_controller/IDLE_AND_TIMER/sim ==

== system npc_controller/CANRX/can_rcv/Switch Case Action Subsystem ==
  Action Port : ActionPort  ActionPortLabel=case [ 10 ]:
  Constant : Constant  OutDataTypeStr=boolean
  Data Store Write : DataStoreWrite  DataStoreName=u8CanDataRx10  IndexOptions=Index vector (dialog)  Indices=1  OutputSizes=1
  Data Store Write1 : DataStoreWrite  DataStoreName=b05_MB10Received  IndexOptions=Index vector (dialog)  Indices=1  OutputSizes=1
  Terminator : Terminator
  eCAN Receive : c280xlib/eCAN Receive  chipFamily=C280x  useModule=eCAN_A  mailboxNo=9  messageID=hex2dec('00000100')  messageType=Standard (11-bit identifier)  enableAcceptanceFiltering=off  messageIDMask=0  sampleTime=-1  dataType=uint8  outputAction=Output last received values  initValue=0  outputMessageID=off  outputMessageLength=off  outputMessageTimeStamp=off  postInterrupt=on  interruptLine=0
      settings: SourceProductBaseCode=TIC2000
  wires:
  eCAN Receive/2 -> Data Store Write/1
  eCAN Receive/1 -> Terminator/1
  Constant/1 -> Data Store Write1/1

== system npc_controller/CANRX/can_rcv/Switch Case Action Subsystem1 ==
  Action Port : ActionPort  ActionPortLabel=case [ 11 ]:
  Constant2 : Constant  OutDataTypeStr=boolean
  Data Store Write1 : DataStoreWrite  DataStoreName=b06_MB11Received  IndexOptions=Index vector (dialog)  Indices=1  OutputSizes=1
  Data Store Write3 : DataStoreWrite  DataStoreName=u8CanDataRx11  IndexOptions=Index vector (dialog)  Indices=1  OutputSizes=1
  Terminator1 : Terminator
  eCAN Receive1 : c280xlib/eCAN Receive  chipFamily=C280x  useModule=eCAN_A  mailboxNo=10  messageID=hex2dec('00000102')  messageType=Standard (11-bit identifier)  enableAcceptanceFiltering=off  messageIDMask=0  sampleTime=-1  dataType=uint8  outputAction=Output last received values  initValue=0  outputMessageID=off  outputMessageLength=off  outputMessageTimeStamp=off  postInterrupt=on  interruptLine=0
      settings: SourceProductBaseCode=TIC2000
  wires:
  eCAN Receive1/1 -> Terminator1/1
  eCAN Receive1/2 -> Data Store Write3/1
  Constant2/1 -> Data Store Write1/1

== system npc_controller/CANRX/can_rcv/Switch Case Action Subsystem2 ==
  Action Port : ActionPort  ActionPortLabel=case [ 12 ]:
  Constant2 : Constant  OutDataTypeStr=boolean
  Data Store Write1 : DataStoreWrite  DataStoreName=u8CanDataRx12  IndexOptions=Index vector (dialog)  Indices=1  OutputSizes=1
  Data Store Write2 : DataStoreWrite  DataStoreName=b07_MB12Received  IndexOptions=Index vector (dialog)  Indices=1  OutputSizes=1
  Terminator2 : Terminator
  eCAN Receive2 : c280xlib/eCAN Receive  chipFamily=C280x  useModule=eCAN_A  mailboxNo=11  messageID=hex2dec('00000108')  messageType=Standard (11-bit identifier)  enableAcceptanceFiltering=off  messageIDMask=0  sampleTime=-1  dataType=uint8  outputAction=Output last received values  initValue=0  outputMessageID=off  outputMessageLength=off  outputMessageTimeStamp=off  postInterrupt=on  interruptLine=0
      settings: SourceProductBaseCode=TIC2000
  wires:
  eCAN Receive2/1 -> Terminator2/1
  eCAN Receive2/2 -> Data Store Write1/1
  Constant2/1 -> Data Store Write2/1

== system npc_controller/CONTROL/CONTROL/false ==
  adc_in : Inport  OutDataTypeStr=Bus: adc_rect
  control_en1 : Inport  Port=2
  ref1 : Inport  Port=3
  angle1 : Inport  Port=4
  pol_pha1 : Inport  Port=5
  pol_phb1 : Inport  Port=6
  pol_phc1 : Inport  Port=7
  pha_en1 : Inport  Port=8
  phb_en1 : Inport  Port=9
  phc_en1 : Inport  Port=10
  pfc_ok2 : Inport  Port=11  OutDataTypeStr=boolean
  Action Port : ActionPort  ActionPortLabel=if(u1 == 0)
  Bus Selector : BusSelector  OutputSignals=va,vb,vc,ia,ib,ic,vbulk,vmid
  CLA Task1 : c2806xlib/CLA Task  taskNumber=1  intSource=Software  wait=off  sampleTime=-1  claType=1  softTrigSelected=1  enableInterrupt=on
      settings: SourceProductBaseCode=TIC2000
  CLA_CONTROL : Subsystem  TreatAsAtomicUnit=on  RTWFcnName=Cla1Task1  RTWFileName=sample_cla
      settings: RTWSystemCode=Inline  RTWFileNameOpts=User specified  RTWMemSecFuncInitTerm=Default  RTWMemSecFuncExecute=Default  RTWMemSecDataInternal=Default
  Variant Sink3 : VariantSink
  sim_cmp1 : Outport
  Vpk : Outport  Port=2
  wires:
  ref1/1 -> CLA_CONTROL/10(ref)
  control_en1/1 -> CLA_CONTROL/9(control_en)
  adc_in/1 -> Bus Selector/1
  pol_phc1/1 -> CLA_CONTROL/14(pol_phc)
  Bus Selector/1 -> CLA_CONTROL/1(va)  "<va>"
  Bus Selector/6 -> CLA_CONTROL/6(ic)  "<ic>"
  angle1/1 -> CLA_CONTROL/11(angle)
  CLA_CONTROL/1(sim_cmp) -> Variant Sink3/1
  Bus Selector/8 -> CLA_CONTROL/8(vmid)  "<vmid>"
  Bus Selector/3 -> CLA_CONTROL/3(vc)  "<vc>"
  Bus Selector/7 -> CLA_CONTROL/7(vbulk)  "<vbulk>"
  Variant Sink3/1 -> sim_cmp1/1
  Bus Selector/4 -> CLA_CONTROL/4(ia)  "<ia>"
  Bus Selector/2 -> CLA_CONTROL/2(vb)  "<vb>"
  CLA Task1/1 -> CLA_CONTROL/Trigger
  Bus Selector/5 -> CLA_CONTROL/5(ib)  "<ib>"
  pol_phb1/1 -> CLA_CONTROL/13(pol_phb)
  pol_pha1/1 -> CLA_CONTROL/12(pol_pha)
  phb_en1/1 -> CLA_CONTROL/16(phb_en1)
  pha_en1/1 -> CLA_CONTROL/15(pha_en1)
  phc_en1/1 -> CLA_CONTROL/17(phc_en1)
  CLA_CONTROL/2(Vpk) -> Vpk/1
  pfc_ok2/1 -> CLA_CONTROL/18(pfc_ok2)

== system npc_controller/CONTROL/GET_ADC/ADC ==
  note: 1) Add Subsystem or Model blocks as valid variant choices.
      | 2) You cannot connect blocks at this level. At simulation, connectivity is automatically
      | determined, based on the active variant and port name matching.
  adc_in : Inport
  codegen : Subsystem  VariantControl=sim_en==false
  sim : Subsystem  VariantControl=sim_en==true
  adc_out : Outport
  adc_rect : Outport  Port=2

== system npc_controller/CONTROL/POLARITY/PLL_Block1 ==
  abc : Inport
  Demux : Demux  Commented=on  Outputs=3
  If1 : If  Commented=on  IfExpression=(u1 > 0)  ShowElse=off
  SRF_PLL : Subsystem
  Subsystem : Subsystem  Commented=on
  theta : Outport  OutDataTypeStr=single
  wires:
  SRF_PLL/3(theta) -> theta/1
  Subsystem/1(Out1) -> If1/1
  abc/1 -> SRF_PLL/1(Vabc), Demux/1
  Demux/1 -> Subsystem/1(In1)

== system npc_controller/CONTROL/STATE-MACHINE/CPU_CONTROL_100_A2_precharge_pfc_ok2/configFutDis ==
  note: Note:
      | TZCCTL
      | 0b00 - High impedance
      | 0b01 - Force to HIGH
      | 0b10 - Force to LOW
      | 0b11 - Do nothing
      |
      | AQCSFRC
      | 0b00 - disables forced PWM
      | 0b01 - forces PWM to LOW
      | 0b10 - forces PWM to  HIGH
  note: /*Force PWM to LOW*/
      | EPwm6Regs.AQCSFRC.bit.CSFA = (uint16_T)(0b01);
      | EPwm6Regs.AQCSFRC.bit.CSFB = (uint16_T)(0b01);
      | EPwm7Regs.AQCSFRC.bit.CSFA = (uint16_T)(0b01);
      | EPwm7Regs.AQCSFRC.bit.CSFB = (uint16_T)(0b01);
      | EPwm8Regs.AQCSFRC.bit.CSFA = (uint16_T)(0b01);
      | EPwm8Regs.AQCSFRC.bit.CSFB = (uint16_T)(0b01);
      | EPwm9Regs.AQCSFRC.bit.CSFA = (uint16_T)(0b01);
      | EPwm9Regs.AQCSFRC.bit.CSFB = (uint16_T)(0b01);
      | EPwm10Regs.AQCSFRC.bit.CSFA = (uint16_T)(0b01);
      | EPwm10Regs.AQCSFRC.bit.CSFB = (uint16_T)(0b01);
      | EPwm11Regs.AQCSFRC.bit.CSFA = (uint16_T)(0b01);
      | EPwm11Regs.AQCSFRC.bit.CSFB = (uint16_T)(0b01);
      |
      | /*Configure TZCTL*/
      | //TZCTL configures TZ action of a DCxEVTy event
      | //0b00=HI-Z, 0b01=HI, 0b10=LO, 0b11=DN
      | EALLOW;
      | EPwm6Regs.TZCTL.bit.DCBEVT1 = 0b10; //LO
      | EPwm6Regs.TZCTL.bit.DCBEVT2 = 0b01; //HI
      | EDIS;
  note: /*Force PWM to LOW*/
      | EPwm2Regs.AQCSFRC.bit.CSFA = (uint16_T)(0b01); force to LOW
      | EPwm2Regs.AQCSFRC.bit.CSFB = (uint16_T)(0b01);
      | EPwm7Regs.AQCSFRC.bit.CSFA = (uint16_T)(0b01);
      | EPwm7Regs.AQCSFRC.bit.CSFB = (uint16_T)(0b01);
      | EPwm8Regs.AQCSFRC.bit.CSFA = (uint16_T)(0b01);
      | EPwm8Regs.AQCSFRC.bit.CSFB = (uint16_T)(0b01);
      | EPwm9Regs.AQCSFRC.bit.CSFA = (uint16_T)(0b01);
      | EPwm9Regs.AQCSFRC.bit.CSFB = (uint16_T)(0b01);
      | EPwm10Regs.AQCSFRC.bit.CSFA = (uint16_T)(0b01);
      | EPwm10Regs.AQCSFRC.bit.CSFB = (uint16_T)(0b01);
      | EPwm11Regs.AQCSFRC.bit.CSFA = (uint16_T)(0b01);
      | EPwm11Regs.AQCSFRC.bit.CSFB = (uint16_T)(0b01);
  f : TriggerPort  TriggerType=function-call  VariantControl=(inherit)
      settings: CopyFcn=Stateflow.SLINSF.SimulinkMan.removeBlockPreDeleteFcn  PreDeleteFcn=Stateflow.SLINSF.SimulinkMan.unsafePredeleteFcn
  System Outputs1 : Subsystem  Commented=on  mask(System Outputs){ShowInLibBrowser=0}
      mask prompts: ShowInLibBrowser "Simulink:masks:CustCodeMaskParam1_MP"
      settings: CopyFcn=cccopyfcn(gcb)  OpenFcn=ccopenfcn('System Outputs Function')
      mask Help: eval('feval(''rtwprivate'',''rtwhelpview'',''rtw_sys_outputs_block'')');
      mask Display: disp('System\nOutputs');
  System Outputs2 : Subsystem  mask(System Outputs){ShowInLibBrowser=0}
      mask prompts: ShowInLibBrowser "Simulink:masks:CustCodeMaskParam1_MP"
      settings: CopyFcn=cccopyfcn(gcb)  OpenFcn=ccopenfcn('System Outputs Function')
      mask Help: eval('feval(''rtwprivate'',''rtwhelpview'',''rtw_sys_outputs_block'')');
      mask Display: disp('System\nOutputs');

== system npc_controller/CONTROL/STATE-MACHINE/CPU_CONTROL_100_A2_precharge_pfc_ok2/configFutEn ==
  note: Note:
      | TZCCTL
      | 0b00 - High impedance
      | 0b01 - Force to HIGH
      | 0b10 - Force to LOW
      | 0b11 - Do nothing
      |
      | AQCSFRC
      | 0b00 - disables forced PWM
      | 0b01 - forces PWM to LOW
      | 0b10 - forces PWM to  HIGH
  note: /*Disable forced PWM*/
      | EPwm2Regs.AQCSFRC.bit.CSFA = (uint16_T)(0b00);
      | EPwm2Regs.AQCSFRC.bit.CSFB = (uint16_T)(0b00);
      | EPwm7Regs.AQCSFRC.bit.CSFA = (uint16_T)(0b00);
      | EPwm7Regs.AQCSFRC.bit.CSFB = (uint16_T)(0b00);
      | EPwm8Regs.AQCSFRC.bit.CSFA = (uint16_T)(0b00);
      | EPwm8Regs.AQCSFRC.bit.CSFB = (uint16_T)(0b00);
      | EPwm9Regs.AQCSFRC.bit.CSFA = (uint16_T)(0b00);
      | EPwm9Regs.AQCSFRC.bit.CSFB = (uint16_T)(0b00);
      | EPwm10Regs.AQCSFRC.bit.CSFA = (uint16_T)(0b00);
      | EPwm10Regs.AQCSFRC.bit.CSFB = (uint16_T)(0b00);
      | EPwm11Regs.AQCSFRC.bit.CSFA = (uint16_T)(0b00);
      | EPwm11Regs.AQCSFRC.bit.CSFB = (uint16_T)(0b00);
      |
      | /*Input unique %duty*/
      | EPwm2Regs.CMPA.bit.CMPA = (uint16_T)(461.4F); //S1
      | EPwm7Regs.CMPB.bit.CMPB = (uint16_T)(461.4F); //S2
      | EPwm2Regs.CMPB.bit.CMPB = (uint16_T)(461.4F); //S3
      | EPwm7Regs.CMPA.bit.CMPA = (uint16_T)(461.4F); //S4
      |
      | EPwm8Regs.CMPB.bit.CMPB = (uint16_T)(922.8F); //S1
      | EPwm9Regs.CMPB.bit.CMPB = (uint16_T)(922.8F); //S2
      | EPwm8Regs.CMPA.bit.CMPA = (uint16_T)(922.8F); //S3
      | EPwm9Regs.CMPA.bit.CMPA = (uint16_T)(922.8F); //S4
      |
      | EPwm10Regs.CMPB.bit.CMPB = (uint16_T)(1384.2F); //S1
      | EPwm11Regs.CMPB.bit.CMPB = (uint16_T)(1384.2F); //S2
      | EPwm10Regs.CMPA.bit.CMPA = (uint16_T)(1384.2F); //S3
      | EPwm11Regs.CMPA.bit.CMPA = (uint16_T)(1384.2F); //S4
  note: //30%duty top cap
      | /*Disable forced PWM*/
      | EPwm6Regs.AQCSFRC.bit.CSFB = (uint16_T)(0b00);
      | EPwm6Regs.AQCSFRC.bit.CSFA = (uint16_T)(0b00);
      | EPwm7Regs.AQCSFRC.bit.CSFA = (uint16_T)(0b01); //LOW
      | EPwm7Regs.AQCSFRC.bit.CSFB = (uint16_T)(0b10); //HIGH
      |
      | EPwm8Regs.AQCSFRC.bit.CSFA = (uint16_T)(0b00);
      | EPwm8Regs.AQCSFRC.bit.CSFB = (uint16_T)(0b00);
      | EPwm9Regs.AQCSFRC.bit.CSFA = (uint16_T)(0b01); //LOW
      | EPwm9Regs.AQCSFRC.bit.CSFB = (uint16_T)(0b10); //HIGH
      |
      | EPwm10Regs.AQCSFRC.bit.CSFA = (uint16_T)(0b00);
      | EPwm10Regs.AQCSFRC.bit.CSFB = (uint16_T)(0b00);
      | EPwm11Regs.AQCSFRC.bit.CSFA = (uint16_T)(0b01); //LOW
      | EPwm11Regs.AQCSFRC.bit.CSFB = (uint16_T)(0b10); //HIGH
      |
      | /*Input unique %duty*/
      | EPwm6Regs.CMPB.bit.CMPB = (uint16_T)(421.4F); //S3
      | EPwm6Regs.CMPA.bit.CMPA = (uint16_T)(501.4F); //S1
      | EPwm7Regs.CMPA.bit.CMPA = (uint16_T)(461.4F); //S4
      | EPwm7Regs.CMPB.bit.CMPB = (uint16_T)(461.4F); //S2
      |
      | EPwm8Regs.CMPA.bit.CMPA = (uint16_T)(421.4F); //S3
      | EPwm8Regs.CMPB.bit.CMPB = (uint16_T)(501.4F); //S1
      | EPwm9Regs.CMPA.bit.CMPA = (uint16_T)(461.4F); //S4
      | EPwm9Regs.CMPB.bit.CMPB = (uint16_T)(461.4F); //S2
      |
      | EPwm10Regs.CMPA.bit.CMPA = (uint16_T)(421.4F); //S3
      | EPwm10Regs.CMPB.bit.CMPB = (uint16_T)(501.4F); //S1
      | EPwm11Regs.CMPA.bit.CMPA = (uint16_T)(461.4F); //S4
      | EPwm11Regs.CMPB.bit.CMPB = (uint16_T)(461.4F); //S2
      |
      | /*Configure TZCTL*/
      | //TZCTL configures TZ action of a DCxEVTy event
      | //0b00=HI-Z, 0b01=HI, 0b10=LO, 0b11=DN
      | EALLOW;
      | EPwm6Regs.TZCTL.bit.DCBEVT1 = 0b11;
      | EPwm6Regs.TZCTL.bit.DCBEVT2 = 0b11;
      | EPwm7Regs.TZCTL.bit.DCBEVT1 = 0b11;
      | EPwm7Regs.TZCTL.bit.DCBEVT2 = 0b11;
      |
      | EPwm8Regs.TZCTL.bit.DCBEVT1 = 0b11;
      | EPwm8Regs.TZCTL.bit.DCBEVT2 = 0b11;
      | EPwm9Regs.TZCTL.bit.DCBEVT1 = 0b11;
      | EPwm9Regs.TZCTL.bit.DCBEVT2 = 0b11;
      |
      | EPwm10Regs.TZCTL.bit.DCBEVT1 = 0b11;
      | EPwm10Regs.TZCTL.bit.DCBEVT2 = 0b11;
      | EPwm11Regs.TZCTL.bit.DCBEVT1 = 0b11;
      | EPwm11Regs.TZCTL.bit.DCBEVT2 = 0b11;
      | EDIS;
  note: //30%duty bot cap
      | /*Disable forced PWM*/
      | EPwm6Regs.AQCSFRC.bit.CSFB = (uint16_T)(0b10); //HIGH
      | EPwm6Regs.AQCSFRC.bit.CSFA = (uint16_T)(0b01); //LOW
      | EPwm7Regs.AQCSFRC.bit.CSFA = (uint16_T)(0b00);
      | EPwm7Regs.AQCSFRC.bit.CSFB = (uint16_T)(0b00);
      |
      | EPwm8Regs.AQCSFRC.bit.CSFA = (uint16_T)(0b10); //HIGH
      | EPwm8Regs.AQCSFRC.bit.CSFB = (uint16_T)(0b01); //LOW
      | EPwm9Regs.AQCSFRC.bit.CSFA = (uint16_T)(0b00);
      | EPwm9Regs.AQCSFRC.bit.CSFB = (uint16_T)(0b00);
      |
      | EPwm10Regs.AQCSFRC.bit.CSFA = (uint16_T)(0b10); //HIGH
      | EPwm10Regs.AQCSFRC.bit.CSFB = (uint16_T)(0b01); //LOW
      | EPwm11Regs.AQCSFRC.bit.CSFA = (uint16_T)(0b00);
      | EPwm11Regs.AQCSFRC.bit.CSFB = (uint16_T)(0b00);
      |
      | /*Input unique %duty*/
      | EPwm6Regs.CMPB.bit.CMPB = (uint16_T)(461.4F); //S3
      | EPwm6Regs.CMPA.bit.CMPA = (uint16_T)(461.4F); //S1
      | EPwm7Regs.CMPA.bit.CMPA = (uint16_T)(501.4F); //S4
      | EPwm7Regs.CMPB.bit.CMPB = (uint16_T)(421.4F); //S2
      |
      | EPwm8Regs.CMPA.bit.CMPA = (uint16_T)(461.4F); //S3
      | EPwm8Regs.CMPB.bit.CMPB = (uint16_T)(461.4F); //S1
      | EPwm9Regs.CMPA.bit.CMPA = (uint16_T)(501.4F); //S4
      | EPwm9Regs.CMPB.bit.CMPB = (uint16_T)(421.4F); //S2
      |
      | EPwm10Regs.CMPA.bit.CMPA = (uint16_T)(461.4F); //S3
      | EPwm10Regs.CMPB.bit.CMPB = (uint16_T)(461.4F); //S1
      | EPwm11Regs.CMPA.bit.CMPA = (uint16_T)(501.4F); //S4
      | EPwm11Regs.CMPB.bit.CMPB = (uint16_T)(421.4F); //S2
      |
      | /*Configure TZCTL*/
      | //TZCTL configures TZ action of a DCxEVTy event
      | //0b00=HI-Z, 0b01=HI, 0b10=LO, 0b11=DN
      | EALLOW;
      | EPwm6Regs.TZCTL.bit.DCBEVT1 = 0b11;
      | EPwm6Regs.TZCTL.bit.DCBEVT2 = 0b11;
      | EPwm7Regs.TZCTL.bit.DCBEVT1 = 0b11;
      | EPwm7Regs.TZCTL.bit.DCBEVT2 = 0b11;
      |
      | EPwm8Regs.TZCTL.bit.DCBEVT1 = 0b11;
      | EPwm8Regs.TZCTL.bit.DCBEVT2 = 0b11;
      | EPwm9Regs.TZCTL.bit.DCBEVT1 = 0b11;
      | EPwm9Regs.TZCTL.bit.DCBEVT2 = 0b11;
      |
      | EPwm10Regs.TZCTL.bit.DCBEVT1 = 0b11;
      | EPwm10Regs.TZCTL.bit.DCBEVT2 = 0b11;
      | EPwm11Regs.TZCTL.bit.DCBEVT1 = 0b11;
      | EPwm11Regs.TZCTL.bit.DCBEVT2 = 0b11;
      | EDIS;
  f : TriggerPort  TriggerType=function-call  VariantControl=(inherit)
      settings: CopyFcn=Stateflow.SLINSF.SimulinkMan.removeBlockPreDeleteFcn  PreDeleteFcn=Stateflow.SLINSF.SimulinkMan.unsafePredeleteFcn
  System Outputs1 : Subsystem  mask(System Outputs){ShowInLibBrowser=0}
      mask prompts: ShowInLibBrowser "Simulink:masks:CustCodeMaskParam1_MP"
      settings: CopyFcn=cccopyfcn(gcb)  OpenFcn=ccopenfcn('System Outputs Function')
      mask Help: eval('feval(''rtwprivate'',''rtwhelpview'',''rtw_sys_outputs_block'')');
      mask Display: disp('System\nOutputs');
  System Outputs2 : Subsystem  Commented=on  mask(System Outputs){ShowInLibBrowser=0}
      mask prompts: ShowInLibBrowser "Simulink:masks:CustCodeMaskParam1_MP"
      settings: CopyFcn=cccopyfcn(gcb)  OpenFcn=ccopenfcn('System Outputs Function')
      mask Help: eval('feval(''rtwprivate'',''rtwhelpview'',''rtw_sys_outputs_block'')');
      mask Display: disp('System\nOutputs');
  System Outputs3 : Subsystem  Commented=on  mask(System Outputs){ShowInLibBrowser=0}
      mask prompts: ShowInLibBrowser "Simulink:masks:CustCodeMaskParam1_MP"
      settings: CopyFcn=cccopyfcn(gcb)  OpenFcn=ccopenfcn('System Outputs Function')
      mask Help: eval('feval(''rtwprivate'',''rtwhelpview'',''rtw_sys_outputs_block'')');
      mask Display: disp('System\nOutputs');
